simulink model "passive_cell_balancing"  (R2021a)
settings: Solver=VariableStepAuto  StartTime=0.0  StopTime=3600  RelTol=1e-3
undefined symbols (not defined in the file): Ion, Lithium
libraries: spsBatteryLib x4, spsMosfetLib x4, spsSeriesRLCBranchLib x4, spspowerguiLib x1
settings Model: Creator=hp  LastModifiedBy=hp

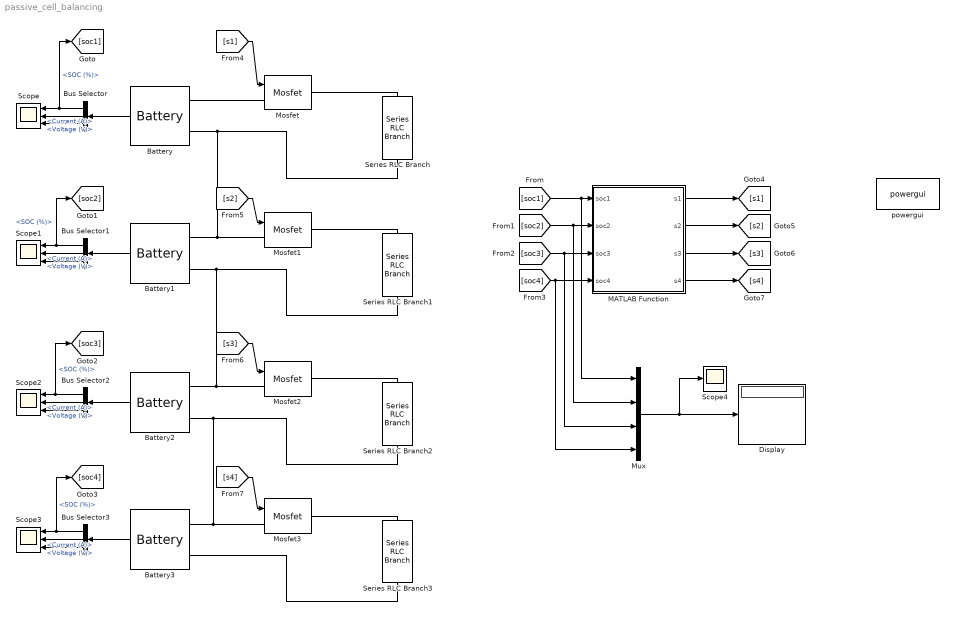
== system passive_cell_balancing ==
  Battery : spsBatteryLib/Battery  BatType=Lithium-Ion  ShowTempParam=off  ThermalPreset=no  ShowAgeParam=off  NomV=3.7  NomQ=2.2  SOC=50  Batt_Tr=30  PresetModel=on  MaxQ=2.2  MinV=2.775  FullV=4.3068  Dis_rate=0.95652  R=0.016818  Normal_OP=1.9896  expZone="[3.9974     0.10809]"  current=[6.5 13 32.5]  Units=Time  Tci=20  NomT=20  T2=-30  MaxQ2=4.8  FullV2=7.1  Normal_OP2=5.655  expZone2="[6.58           1]"  Rca=0.6  ti=2000  Dp=0  Neq0=0  Tsim=1e6  Ta1=25  Qeol=5.4*0.9  Reol=0.013333*1.2  Char_age=[2.3478, 3]  Dis_age=[2.3478, 10]  N1=1500  N2=10500  N3=1000  N4=1400  Ta2=45  N5=950
  Battery1 : spsBatteryLib/Battery  BatType=Lithium-Ion  ShowTempParam=off  ThermalPreset=no  ShowAgeParam=off  NomV=3.7  NomQ=2.2  SOC=45  Batt_Tr=30  PresetModel=on  MaxQ=2.2  MinV=2.775  FullV=4.3068  Dis_rate=0.95652  R=0.016818  Normal_OP=1.9896  expZone="[3.9974     0.10809]"  current=[6.5 13 32.5]  Units=Time  Tci=20  NomT=20  T2=-30  MaxQ2=4.8  FullV2=7.1  Normal_OP2=5.655  expZone2="[6.58           1]"  Rca=0.6  ti=2000  Dp=0  Neq0=0  Tsim=1e6  Ta1=25  Qeol=5.4*0.9  Reol=0.013333*1.2  Char_age=[2.3478, 3]  Dis_age=[2.3478, 10]  N1=1500  N2=10500  N3=1000  N4=1400  Ta2=45  N5=950
  Battery2 : spsBatteryLib/Battery  BatType=Lithium-Ion  ShowTempParam=off  ThermalPreset=no  ShowAgeParam=off  NomV=3.7  NomQ=2.2  SOC=55  Batt_Tr=30  PresetModel=on  MaxQ=2.2  MinV=2.775  FullV=4.3068  Dis_rate=0.95652  R=0.016818  Normal_OP=1.9896  expZone="[3.9974     0.10809]"  current=[6.5 13 32.5]  Units=Time  Tci=20  NomT=20  T2=-30  MaxQ2=4.8  FullV2=7.1  Normal_OP2=5.655  expZone2="[6.58           1]"  Rca=0.6  ti=2000  Dp=0  Neq0=0  Tsim=1e6  Ta1=25  Qeol=5.4*0.9  Reol=0.013333*1.2  Char_age=[2.3478, 3]  Dis_age=[2.3478, 10]  N1=1500  N2=10500  N3=1000  N4=1400  Ta2=45  N5=950
  Battery3 : spsBatteryLib/Battery  BatType=Lithium-Ion  ShowTempParam=off  ThermalPreset=no  ShowAgeParam=off  NomV=3.7  NomQ=2.2  SOC=58  Batt_Tr=30  PresetModel=on  MaxQ=2.2  MinV=2.775  FullV=4.3068  Dis_rate=0.95652  R=0.016818  Normal_OP=1.9896  expZone="[3.9974     0.10809]"  current=[6.5 13 32.5]  Units=Time  Tci=20  NomT=20  T2=-30  MaxQ2=4.8  FullV2=7.1  Normal_OP2=5.655  expZone2="[6.58           1]"  Rca=0.6  ti=2000  Dp=0  Neq0=0  Tsim=1e6  Ta1=25  Qeol=5.4*0.9  Reol=0.013333*1.2  Char_age=[2.3478, 3]  Dis_age=[2.3478, 10]  N1=1500  N2=10500  N3=1000  N4=1400  Ta2=45  N5=950
  Bus Selector{,1..3} (4 alike) : BusSelector  OutputSignals=SOC (%),Current (A),Voltage (V)
  Display : Display
  MATLAB Function : MATLAB Function  TreatAsAtomicUnit=on
  Mosfet{,1..3} (4 alike) : spsMosfetLib/Mosfet  Ron=0.1  Lon=0  Rd=0.01  Vfd=0  IC=0  Rs=1e5  Cs=inf  Measurements=off
  Mux : Mux
  Scope{,1..3} (4 alike) : Scope  NumInputPorts=3
  Scope4 : Scope
  Series RLC Branch{,1..3} (4 alike) : spsSeriesRLCBranchLib/Series RLC Branch  LConnTagsString=__new0  RConnTagsString=__new0  BranchType=R  Resistance=1  Inductance=1e-3  SetiL0=off  InitialCurrent=0  Capacitance=1e-6  Setx0=off  InitialVoltage=0  Measurements=None
  powergui : spspowerguiLib/powergui  Priority=1  SimulationMode=Discrete  SampleTime=10e-3  frequency=60  Iterations=50  frequencyindice=0  Pbase=100e6  ErrMax=1e-4  UnitsV=kV  UnitsW=MW  buscounter=0  FunctionMessages=off  echomessages=off  EnableUseOfTLC=off  CurrentSourceSwitches=off  DisableSnubberDevices=off  DisableRonSwitches=off  DisableVfSwitches=off  DisplayEquations=off  AutomaticDiscreteSolvers=off  SolverType=Tustin/Backward Euler (TBE)  Interpol=off  ExternalGateDelay=off  methode=off  Ts=100  x0status=blocks  SPID=on  SwTol=0  HookPort=off  NonlinearTolerance=1e-4  nMaxIteration=100  ContinueOnMaxIteration=off  RestoreLinks=warning  ResistiveCurrentMeasurement=off  Frange=[0:2:500]  Ylog=off  Xlog=on  ShowGrid=off  save=off  variable=ZData  structure=0  ZoomFFT=off  StartTime=0.0  cycles=1  DisplayStyle=1  fundamental=60  FreqAxis=off  MaxFrequency=1000  frequencyindicesteady=1  RmsSteady=1  display=off
  wires:
  Battery/1 -> Bus Selector/1
  Bus Selector/1 -> [soc1], Scope/1  "<SOC (%)>"
  Bus Selector/2 -> Scope/2  "<Current (A)>"
  Bus Selector/3 -> Scope/3  "<Voltage (V)>"
  Bus Selector1/3 -> Scope1/3  "<Voltage (V)>"
  Bus Selector1/2 -> Scope1/2  "<Current (A)>"
  Bus Selector1/1 -> [soc2], Scope1/1  "<SOC (%)>"
  Battery1/1 -> Bus Selector1/1
  Battery3/1 -> Bus Selector3/1
  Bus Selector3/1 -> [soc4], Scope3/1  "<SOC (%)>"
  Bus Selector3/2 -> Scope3/2  "<Current (A)>"
  Bus Selector3/3 -> Scope3/3  "<Voltage (V)>"
  Bus Selector2/3 -> Scope2/3  "<Voltage (V)>"
  Bus Selector2/2 -> Scope2/2  "<Current (A)>"
  Bus Selector2/1 -> [soc3], Scope2/1  "<SOC (%)>"
  Battery2/1 -> Bus Selector2/1
  [soc1] -> Mux/1, MATLAB Function/1(soc1)
  [soc2] -> MATLAB Function/2(soc2), Mux/2
  [soc3] -> MATLAB Function/3(soc3), Mux/3
  [soc4] -> MATLAB Function/4(soc4), Mux/4
  MATLAB Function/4(s4) -> [s4]
  MATLAB Function/3(s3) -> [s3]
  MATLAB Function/2(s2) -> [s2]
  MATLAB Function/1(s1) -> [s1]
  [s1] -> Mosfet/1
  [s2] -> Mosfet1/1
  [s3] -> Mosfet2/1
  [s4] -> Mosfet3/1
  Mux/1 -> Scope4/1, Display/1
  connections:
  Mosfet/LConn1 -- Battery/LConn1
  Mosfet/RConn1 -- Series RLC Branch/LConn1
  Mosfet1/RConn1 -- Series RLC Branch1/LConn1
  Series RLC Branch/RConn1 -- Battery1/LConn1 -- Mosfet1/LConn1 -- Battery/LConn2
  Series RLC Branch2/RConn1 -- Battery3/LConn1 -- Mosfet3/LConn1 -- Battery2/LConn2
  Mosfet3/RConn1 -- Series RLC Branch3/LConn1
  Mosfet2/RConn1 -- Series RLC Branch2/LConn1
  Series RLC Branch3/RConn1 -- Battery3/LConn2
  Series RLC Branch1/RConn1 -- Battery2/LConn1 -- Mosfet2/LConn1 -- Battery1/LConn2

== matlab function passive_cell_balancing/MATLAB Function ==
  data: soc1 input; s1 output; soc2 input; soc3 input; soc4 input; s2 output; s3 output; s4 output
function [s1,s2,s3,s4] = fcn(soc1, soc2, soc3, soc4)
soc1=int64(soc1);
soc2=int64(soc2);
soc3=int64(soc3);
soc4=int64(soc4);

if((soc1>soc2)||(soc1>soc3)||(soc1>soc4))
    s1=1;
else
    s1=0;
end
if((soc2>soc1)||(soc2>soc3)||(soc2>soc4))
    s2=1;
else
    s2=0;
end
if((soc3>soc1)||(soc3>soc2)||(soc3>soc4))
    s3=1;
else
    s3=0;
end
if((soc4>soc1)||(soc4>soc2)||(soc4>soc3))
    s4=1;
else
    s4=0;
end
